simulink model "Target_Control_System"  (R2021b)
settings: Solver=FixedStepDiscrete  StartTime=0.0  StopTime=5  RelTol=1e-3
PreLoadFcn:
  | RTWConfigurationCB('preloadfcn', bdroot);
PostLoadFcn:
  | load('configuration/data_struct.mat');
  | load('configuration/fluxMaps_propMotor.mat');
  | load('configuration/parameterInit_PROP.mat');
  | load('configuration/parameterInit_PUMP.mat');
  | load('configuration/parameterInit_PITCH.mat');
  | load('configuration/parameterInit_TILT.mat');
  | %load('configuration/base_workspace_signal_definition.mat');
  | %load('resolvedatastores_to_baseworkspace_for_faster_simulation.mat');
model workspace (MAT data in the model file):
  SIMULATION_OPTIONS : Simulink.Parameter (value not decoded)
  TARGET_CODE_GEN : Simulink.Parameter (value not decoded)
  TCS_SAMPLE_FREQ_HZ : Simulink.Parameter (value not decoded)
symbols that are objects in the model workspace (value not decoded): TARGET_CODE_GEN, TCS_SAMPLE_FREQ_HZ
undefined symbols (not defined in the file): A_DQ_REF_LPF_INIT__PITCH, A_DQ_REF_LPF_INIT__PROP, A_DQ_REF_LPF_INIT__PUMP, A_DQ_REF_LPF_INIT__TILT, A_OBSERVER_CONFIDENCE_INIT__PITCH, A_OBSERVER_CONFIDENCE_INIT__PROP, A_OBSERVER_CONFIDENCE_INIT__PUMP, A_OBSERVER_CONFIDENCE_INIT__TILT, ACTUATOR_MAX_ANGLE_TRIP__PITCH, ACTUATOR_MIN_ANGLE_TRIP__PITCH, ACTUATOR_POS_SENSOR_INV_DIRECTION__PITCH, ACTUATOR_POS_SENSOR_INV_DIRECTION__TILT, ACTUATOR_POS_SENSOR_OFFSET__PITCH, ACTUATOR_POS_SENSOR_OFFSET__TILT, ADC_scaler1_baseaddr_TILT, ADC_SCALER_FLOAT_TO_FIXPOINT_EXPANSION, ANGLE_ELEC_FROM_SENSOR_OFFSET_INIT__PITCH, ANGLE_ELEC_FROM_SENSOR_OFFSET_INIT__PROP, ANGLE_ELEC_FROM_SENSOR_OFFSET_INIT__PUMP, ANGLE_ELEC_FROM_SENSOR_OFFSET_INIT__TILT, AUTO_CLEAR_FAULTS_ENABLED__PITCH, AUTO_CLEAR_FAULTS_ENABLED__PROP, AUTO_CLEAR_FAULTS_ENABLED__PUMP, AUTO_CLEAR_FAULTS_ENABLED__TILT, AUTO_CLEAR_FAULTS_WAIT_TICKS__PITCH, AUTO_CLEAR_FAULTS_WAIT_TICKS__PROP, AUTO_CLEAR_FAULTS_WAIT_TICKS__PUMP, AUTO_CLEAR_FAULTS_WAIT_TICKS__TILT, AUTO_I_ZERO_IDLE_TICKS__PITCH, AUTO_I_ZERO_IDLE_TICKS__PROP, AUTO_I_ZERO_IDLE_TICKS__PUMP, AUTO_I_ZERO_IDLE_TICKS__TILT, AUTO_I_ZERO_OFFSET_IDC_THRESHOLD__PITCH, AUTO_I_ZERO_OFFSET_IDC_THRESHOLD__PROP, AUTO_I_ZERO_OFFSET_IDC_THRESHOLD__PUMP, AUTO_I_ZERO_OFFSET_IDC_THRESHOLD__TILT, AUTO_I_ZERO_OFFSET_IPH_THRESHOLD__PITCH, AUTO_I_ZERO_OFFSET_IPH_THRESHOLD__PROP, AUTO_I_ZERO_OFFSET_IPH_THRESHOLD__PUMP, AUTO_I_ZERO_OFFSET_IPH_THRESHOLD__TILT, AUTO_SENSORLESS_SWITCHOVER_DISABLE_OMEGA, AUTO_SENSORLESS_SWITCHOVER_ENABLE_OMEGA, AUTO_SENSORLESS_SWITCHOVER_MIN_CONFIDENCE, AUXILIARY_PROTECTION_UNIT_BASEADDR__TILT, blanking_max_error_omega_INIT_PITCH, blanking_max_error_omega_INIT_TILT, blanking_max_error_position_INIT_PITCH, blanking_max_error_position_INIT_TILT, BRUTE_START_I_Q_REF_RAMP_SPEED__PITCH, BRUTE_START_I_Q_REF_RAMP_SPEED__PROP, BRUTE_START_I_Q_REF_RAMP_SPEED__PUMP, BRUTE_START_I_Q_REF_RAMP_SPEED__TILT, CONTROL_LOOP_DT_INIT__PITCH, CONTROL_LOOP_DT_INIT__PROP, CONTROL_LOOP_DT_INIT__PUMP, CONTROL_LOOP_DT_INIT__TILT, CORRECTION_FILTER_SCALE__PITCH, CORRECTION_FILTER_SCALE__PROP, CORRECTION_FILTER_SCALE__PUMP, CORRECTION_FILTER_SCALE__TILT ... (+458)
libraries: simulink x178, Reusables_Lib x24
(part 32 of 47)

== system Target_Control_System/Target_Control_System/Simulation Controls/Simulation Data Store Initialization/setupPwm()/setPwmFrequencyApplication()_pitch/updateObserver()_pitch ==
  oIsr_.oParam_.fControlLoopDt_ : Inport
  fObserverLoopFilterBandwidthHz_ : Inport  Port=2
  Constant : Constant  Value=15*2*pi  OutDataTypeStr=single  SampleTime=-1
  Constant1 : Constant  Value=8*2*pi  OutDataTypeStr=single  SampleTime=-1
  Constant2 : Constant  Value=2*pi  OutDataTypeStr=single  SampleTime=-1
  Constant3 : Constant  Value=500  OutDataTypeStr=single  SampleTime=-1
  Constant4 : Constant  Value=20  OutDataTypeStr=single  SampleTime=-1
  Constant5 : Constant  Value=100*2*pi  OutDataTypeStr=single  SampleTime=-1
  Constant6 : Constant  Value=4*2*pi  OutDataTypeStr=single  SampleTime=-1
  Constant7 : Constant  Value=0.0625  OutDataTypeStr=single  SampleTime=-1
  Data Store Write : DataStoreWrite  DataStoreName=oPitch  DataStoreElements=oPitch.oIsr_.oParam_.fALpf4hpfDcBlocking_  IndexOptions=Index vector (dialog)  Indices=1  OutputSizes=1
  Data Store Write1 : DataStoreWrite  DataStoreName=oPitch  DataStoreElements=oPitch.oIsr_.oParam_.fAFluxMagnitude_  IndexOptions=Index vector (dialog)  Indices=1  OutputSizes=1
  Data Store Write2 : DataStoreWrite  DataStoreName=oPitch  DataStoreElements=oPitch.oIsr_.oParam_.fALoopfilter2_  IndexOptions=Index vector (dialog)  Indices=1  OutputSizes=1
  Data Store Write3 : DataStoreWrite  DataStoreName=oPitch  DataStoreElements=oPitch.oMot_.oParam_.fObserverLoopFilterBandwidthHz_  IndexOptions=Index vector (dialog)  Indices=1  OutputSizes=1
  Data Store Write4 : DataStoreWrite  DataStoreName=oPitch  DataStoreElements=oPitch.oIsr_.oParam_.fAOmegaFilter2_  IndexOptions=Index vector (dialog)  Indices=1  OutputSizes=1
  Data Store Write5 : DataStoreWrite  DataStoreName=oPitch  DataStoreElements=oPitch.oMot_.oParam_.fAOmegaXfilter2_  IndexOptions=Index vector (dialog)  Indices=1  OutputSizes=1
  Data Store Write6 : DataStoreWrite  DataStoreName=oPitch  DataStoreElements=oPitch.oIsr_.oParam_.oPiDataPll2_.oParameter_.fKp_  IndexOptions=Index vector (dialog)  Indices=1  OutputSizes=1
  Divide{,1,3..4} (4 alike) : Product  Inputs=**
  Divide2 : Product  Inputs=***
  Divide5 : Product  Inputs=*/
  GreaterThan : RelationalOperator  Operator=<  OutDataTypeStr=boolean  RndMeth=Simplest
  Saturation{,1..4} (5 alike) : Saturate  UpperLimit=1.0  LowerLimit=1e-6
  Switch : Switch  Criteria=u2 > Threshold
  wires:
  Divide5/1 -> Data Store Write6/1
  Constant7/1 -> Divide5/1
  Saturation4/1 -> Data Store Write5/1
  oIsr_.oParam_.fControlLoopDt_/1 -> Divide/1, Divide1/1, Divide3/1, Divide2/2, Divide5/2, Divide4/1
  Divide4/1 -> Saturation4/1
  Constant6/1 -> Divide4/2
  Saturation3/1 -> Data Store Write4/1
  Divide3/1 -> Saturation3/1
  Constant5/1 -> Divide3/2
  Switch/1 -> Data Store Write3/1, Divide2/1
  Constant3/1 -> Switch/1
  GreaterThan/1 -> Switch/2
  Constant4/1 -> GreaterThan/2
  fObserverLoopFilterBandwidthHz_/1 -> Switch/3, GreaterThan/1
  Divide2/1 -> Saturation2/1
  Saturation2/1 -> Data Store Write2/1
  Constant2/1 -> Divide2/3
  Divide1/1 -> Saturation1/1
  Saturation1/1 -> Data Store Write1/1
  Constant1/1 -> Divide1/2
  Saturation/1 -> Data Store Write/1
  Divide/1 -> Saturation/1
  Constant/1 -> Divide/2

== system Target_Control_System/Target_Control_System/Simulation Controls/Simulation Data Store Initialization/updateServoObserver(&oTilt)/updateServoObserver()/softwareIirFilterInitialize() ==
  fFreq3db : Inport
  fFreqSample : Inport  Port=2  OutDataTypeStr=single
  Constant : Constant  OutDataTypeStr=single  SampleTime=-1
  Constant1 : Constant  Value=0  OutDataTypeStr=single  SampleTime=-1
  Data Store Write : DataStoreWrite  DataStoreName=oTilt  DataStoreElements=oTilt.oMot_.oState_.oPosSensor_.oInputSensorSpeedFilter_.afConstantsA_.h0  IndexOptions=Index vector (dialog)  Indices=1  OutputSizes=1
  Data Store Write1 : DataStoreWrite  DataStoreName=oTilt  DataStoreElements=oTilt.oMot_.oState_.oPosSensor_.oInputSensorSpeedFilter_.afConstantsA_.h1  IndexOptions=Index vector (dialog)  Indices=1  OutputSizes=1
  Data Store Write10 : DataStoreWrite  DataStoreName=oTilt  DataStoreElements=oTilt.oMot_.oState_.oPosSensor_.oInputSensorSpeedFilter_.fFilterOutput_  IndexOptions=Index vector (dialog)  Indices=1  OutputSizes=1
  Data Store Write2 : DataStoreWrite  DataStoreName=oTilt  DataStoreElements=oTilt.oMot_.oState_.oPosSensor_.oInputSensorSpeedFilter_.afConstantsA_.h2  IndexOptions=Index vector (dialog)  Indices=1  OutputSizes=1
  Data Store Write3 : DataStoreWrite  DataStoreName=oTilt  DataStoreElements=oTilt.oMot_.oState_.oPosSensor_.oInputSensorSpeedFilter_.afConstantsB_.h2  IndexOptions=Index vector (dialog)  Indices=1  OutputSizes=1
  Data Store Write4 : DataStoreWrite  DataStoreName=oTilt  DataStoreElements=oTilt.oMot_.oState_.oPosSensor_.oInputSensorSpeedFilter_.afConstantsB_.h1  IndexOptions=Index vector (dialog)  Indices=1  OutputSizes=1
  Data Store Write5 : DataStoreWrite  DataStoreName=oTilt  DataStoreElements=oTilt.oMot_.oState_.oPosSensor_.oInputSensorSpeedFilter_.afConstantsB_.h0  IndexOptions=Index vector (dialog)  Indices=1  OutputSizes=1
  Data Store Write6 : DataStoreWrite  DataStoreName=oTilt  DataStoreElements=oTilt.oMot_.oState_.oPosSensor_.oInputSensorSpeedFilter_.afPreviousInputs_.h0  IndexOptions=Index vector (dialog)  Indices=1  OutputSizes=1
  Data Store Write7 : DataStoreWrite  DataStoreName=oTilt  DataStoreElements=oTilt.oMot_.oState_.oPosSensor_.oInputSensorSpeedFilter_.afPreviousInputs_.h1  IndexOptions=Index vector (dialog)  Indices=1  OutputSizes=1
  Data Store Write8 : DataStoreWrite  DataStoreName=oTilt  DataStoreElements=oTilt.oMot_.oState_.oPosSensor_.oInputSensorSpeedFilter_.afPreviousOutputs_.h0  IndexOptions=Index vector (dialog)  Indices=1  OutputSizes=1
  Data Store Write9 : DataStoreWrite  DataStoreName=oTilt  DataStoreElements=oTilt.oMot_.oState_.oPosSensor_.oInputSensorSpeedFilter_.afPreviousOutputs_.h1  IndexOptions=Index vector (dialog)  Indices=1  OutputSizes=1
  Data Type Conversion{,1..4} (5 alike) : DataTypeConversion  OutDataTypeStr=single
  Demux : Demux  Outputs=6
  Divide : Product  Inputs=*/  OutDataTypeStr=single
  computeCoefficientsButter() : Subsystem
  fActualFrequencyHz : Outport
  wires:
  fFreqSample/1 -> computeCoefficientsButter()/2(dSampleFrequencyHz)
  Data Type Conversion4/1 -> Data Store Write2/1
  Data Type Conversion3/1 -> Data Store Write1/1
  Data Type Conversion2/1 -> Data Store Write3/1
  Data Type Conversion/1 -> Data Store Write4/1
  Data Type Conversion1/1 -> Data Store Write5/1
  Constant1/1 -> Data Store Write6/1, Data Store Write7/1, Data Store Write9/1, Data Store Write10/1, Data Store Write8/1
  Demux/1 -> Data Type Conversion1/1
  Demux/2 -> Data Type Conversion/1
  Constant/1 -> Divide/1
  Divide/1 -> Data Store Write/1
  Demux/4 -> Divide/2
  Demux/3 -> Data Type Conversion2/1
  Demux/5 -> Data Type Conversion3/1
  Demux/6 -> Data Type Conversion4/1
  computeCoefficientsButter()/1(dpOutArray) -> Demux/1
  fFreq3db/1 -> computeCoefficientsButter()/1(fCutoffFrequencyHz)
  computeCoefficientsButter()/2(fFreq3db) -> fActualFrequencyHz/1

== system Target_Control_System/Target_Control_System/Simulation Controls/Simulation Data Store Initialization/updateServoObserver()/updateServoObserver()_pitch/softwareIirFilterInitialize() ==
  fFreq3db : Inport
  fFreqSample : Inport  Port=2  OutDataTypeStr=single
  Constant : Constant  OutDataTypeStr=single  SampleTime=-1
  Constant1 : Constant  Value=0  OutDataTypeStr=single  SampleTime=-1
  Data Store Write : DataStoreWrite  DataStoreName=oPitch  DataStoreElements=oPitch.oMot_.oState_.oPosSensor_.oInputSensorSpeedFilter_.afConstantsA_.h0  IndexOptions=Index vector (dialog)  Indices=1  OutputSizes=1
  Data Store Write1 : DataStoreWrite  DataStoreName=oPitch  DataStoreElements=oPitch.oMot_.oState_.oPosSensor_.oInputSensorSpeedFilter_.afConstantsA_.h1  IndexOptions=Index vector (dialog)  Indices=1  OutputSizes=1
  Data Store Write10 : DataStoreWrite  DataStoreName=oPitch  DataStoreElements=oPitch.oMot_.oState_.oPosSensor_.oInputSensorSpeedFilter_.fFilterOutput_  IndexOptions=Index vector (dialog)  Indices=1  OutputSizes=1
  Data Store Write2 : DataStoreWrite  DataStoreName=oPitch  DataStoreElements=oPitch.oMot_.oState_.oPosSensor_.oInputSensorSpeedFilter_.afConstantsA_.h2  IndexOptions=Index vector (dialog)  Indices=1  OutputSizes=1
  Data Store Write3 : DataStoreWrite  DataStoreName=oPitch  DataStoreElements=oPitch.oMot_.oState_.oPosSensor_.oInputSensorSpeedFilter_.afConstantsB_.h2  IndexOptions=Index vector (dialog)  Indices=1  OutputSizes=1
  Data Store Write4 : DataStoreWrite  DataStoreName=oPitch  DataStoreElements=oPitch.oMot_.oState_.oPosSensor_.oInputSensorSpeedFilter_.afConstantsB_.h1  IndexOptions=Index vector (dialog)  Indices=1  OutputSizes=1
  Data Store Write5 : DataStoreWrite  DataStoreName=oPitch  DataStoreElements=oPitch.oMot_.oState_.oPosSensor_.oInputSensorSpeedFilter_.afConstantsB_.h0  IndexOptions=Index vector (dialog)  Indices=1  OutputSizes=1
  Data Store Write6 : DataStoreWrite  DataStoreName=oPitch  DataStoreElements=oPitch.oMot_.oState_.oPosSensor_.oInputSensorSpeedFilter_.afPreviousInputs_.h0  IndexOptions=Index vector (dialog)  Indices=1  OutputSizes=1
  Data Store Write7 : DataStoreWrite  DataStoreName=oPitch  DataStoreElements=oPitch.oMot_.oState_.oPosSensor_.oInputSensorSpeedFilter_.afPreviousInputs_.h1  IndexOptions=Index vector (dialog)  Indices=1  OutputSizes=1
  Data Store Write8 : DataStoreWrite  DataStoreName=oPitch  DataStoreElements=oPitch.oMot_.oState_.oPosSensor_.oInputSensorSpeedFilter_.afPreviousOutputs_.h0  IndexOptions=Index vector (dialog)  Indices=1  OutputSizes=1
  Data Store Write9 : DataStoreWrite  DataStoreName=oPitch  DataStoreElements=oPitch.oMot_.oState_.oPosSensor_.oInputSensorSpeedFilter_.afPreviousOutputs_.h1  IndexOptions=Index vector (dialog)  Indices=1  OutputSizes=1
  Data Type Conversion{,1..4} (5 alike) : DataTypeConversion  OutDataTypeStr=single
  Demux : Demux  Outputs=6
  Divide : Product  Inputs=*/  OutDataTypeStr=single
  computeCoefficientsButter() : Subsystem
  fActualFrequencyHz : Outport
  wires:
  fFreqSample/1 -> computeCoefficientsButter()/2(dSampleFrequencyHz)
  Data Type Conversion4/1 -> Data Store Write2/1
  Data Type Conversion3/1 -> Data Store Write1/1
  Data Type Conversion2/1 -> Data Store Write3/1
  Data Type Conversion/1 -> Data Store Write4/1
  Data Type Conversion1/1 -> Data Store Write5/1
  Constant1/1 -> Data Store Write6/1, Data Store Write7/1, Data Store Write9/1, Data Store Write10/1, Data Store Write8/1
  Demux/1 -> Data Type Conversion1/1
  Demux/2 -> Data Type Conversion/1
  Constant/1 -> Divide/1
  Divide/1 -> Data Store Write/1
  Demux/4 -> Divide/2
  Demux/3 -> Data Type Conversion2/1
  Demux/5 -> Data Type Conversion3/1
  Demux/6 -> Data Type Conversion4/1
  computeCoefficientsButter()/1(dpOutArray) -> Demux/1
  fFreq3db/1 -> computeCoefficientsButter()/1(fCutoffFrequencyHz)
  computeCoefficientsButter()/2(fFreq3db) -> fActualFrequencyHz/1

== system Target_Control_System/Target_Control_System/InterruptFunction/pitchMotor_dataToMain/Variant Subsystem/VP_leader_follower_postion_copy/Follower Postion Enabled Subsystem/System Update ==

== system Target_Control_System/Target_Control_System/InterruptFunction/pitchMotor_dataToMain/Variant Subsystem/VP_leader_follower_postion_copy/Leader Postion Enabled Subsystem/System Update ==

== system Target_Control_System/Target_Control_System/InterruptFunction/pitchMotor_isrTask/abcToAlphaBeta/ModelSource/IncludeCustomCode/System Update ==

== system Target_Control_System/Target_Control_System/InterruptFunction/pitchMotor_isrTask/currentController/Current Controller/Limit Voltage Vector/Compute Alpha-Beta Refs ==
  In1 : Inport
  Out1 : Outport
  wires:
  In1/1 -> Out1/1

== system Target_Control_System/Target_Control_System/InterruptFunction/pitchMotor_isrTask/fluxAngleCalculations/ModelSource/IncludeCustomCode/System Update ==

== system Target_Control_System/Target_Control_System/InterruptFunction/propMotor_isrTask/abcToAlphaBeta/ModelSourceFOProp/IncludeCustomCode/System Update ==

== system Target_Control_System/Target_Control_System/InterruptFunction/propMotor_isrTask/currentController/Subsystem/Limit Voltage Vector/Subsystem ==
  fMaximumVoltageVectorLengthSquared_ : Inport
  UdRef*UdRef : Inport  Port=2
  In3 : Inport  Port=3
  Enable : EnablePort
  Add1 : Sum  Inputs=+-
  Constant1 : Constant  Value=0  OutDataTypeStr=single  SampleTime=-1
  Divide3 : Product  Inputs=**
  Max : MinMax  Function=max  Inputs=2
  Sqrt : Sqrt  SaturateOnIntegerOverflow=on
  Out1 : Outport
  wires:
  UdRef*UdRef/1 -> Add1/2
  fMaximumVoltageVectorLengthSquared_/1 -> Add1/1
  Divide3/1 -> Out1/1
  Add1/1 -> Max/2
  Constant1/1 -> Max/1
  Max/1 -> Sqrt/1
  In3/1 -> Divide3/2
  Sqrt/1 -> Divide3/1

== system Target_Control_System/Target_Control_System/InterruptFunction/propMotor_isrTask/fluxAngleCalculation/ModelSource/IncludeCustomCode/System Update ==

== system Target_Control_System/Target_Control_System/InterruptFunction/pumpMotor_isrTask/abcToAlphaBeta/ModelSource/IncludeCustomCode/System Update ==

== system Target_Control_System/Target_Control_System/InterruptFunction/pumpMotor_isrTask/currentController/Subsystem/Limit Voltage Vector/Subsystem ==
  fMaximumVoltageVectorLengthSquared_ : Inport
  UdRef*UdRef : Inport  Port=2
  In3 : Inport  Port=3
  Enable : EnablePort
  Add1 : Sum  Inputs=+-
  Constant1 : Constant  Value=0  OutDataTypeStr=single  SampleTime=-1
  Divide3 : Product  Inputs=**
  Max : MinMax  Function=max  Inputs=2
  Sqrt : Sqrt  SaturateOnIntegerOverflow=on
  Out1 : Outport
  wires:
  UdRef*UdRef/1 -> Add1/2
  fMaximumVoltageVectorLengthSquared_/1 -> Add1/1
  Divide3/1 -> Out1/1
  Add1/1 -> Max/2
  Constant1/1 -> Max/1
  Max/1 -> Sqrt/1
  In3/1 -> Divide3/2
  Sqrt/1 -> Divide3/1

== system Target_Control_System/Target_Control_System/InterruptFunction/pumpMotor_isrTask/fluxAngleCalculations/ModelSource1/IncludeCustomCode/System Update ==

== system Target_Control_System/Target_Control_System/InterruptFunction/tiltMotor_isrTask/abcToAlphaBeta/ModelSource/IncludeCustomCode/System Update ==

== system Target_Control_System/Target_Control_System/InterruptFunction/tiltMotor_isrTask/currentController/Enabled Subsystem/Limit Voltage Vector/Compute Alpha-Beta Refs ==
  In1 : Inport
  Out1 : Outport
  wires:
  In1/1 -> Out1/1

== system Target_Control_System/Target_Control_System/InterruptFunction/tiltMotor_isrTask/fluxAngleCalculation/ModelSource/IncludeCustomCode/System Update ==

== system Target_Control_System/Target_Control_System/MainLoop/pitchMotor_mainLoop/Decimation gate for 10 Hz Pitch/Function-Call Subsystem/Dynamic_current_limiting_pitch/Enabled Subsystem ==
  Enable : EnablePort
  Constant : Constant  Value=0  OutDataTypeStr=single  SampleTime=-1
  Constant1 : Constant  Value=200  OutDataTypeStr=single  SampleTime=-1
  Constant3 : Constant  Value=0  OutDataTypeStr=single  SampleTime=-1
  Data Store Read : DataStoreRead  DataStoreName=oPitch  DataStoreElements=oPitch.oMot_.oParam_.fDynILimDynamicMax_  IndexOptions=Index vector (dialog)  Indices=1  OutputSizes=1
  Data Store Read1 : DataStoreRead  DataStoreName=oPitch  DataStoreElements=oPitch.oMot_.oParam_.fDynILimKnockdownFactor_  IndexOptions=Index vector (dialog)  Indices=1  OutputSizes=1
  Data Store Read2 : DataStoreRead  DataStoreName=oPitch  DataStoreElements=oPitch.oMot_.oParam_.fDynILimDynamicMax_  IndexOptions=Index vector (dialog)  Indices=1  OutputSizes=1
  Data Store Read3 : DataStoreRead  DataStoreName=oPitch  DataStoreElements=oPitch.oMot_.oState_.fDynILimIntegrator_  IndexOptions=Index vector (dialog)  Indices=1  OutputSizes=1
  Data Store Read4 : DataStoreRead  DataStoreName=oPitch  DataStoreElements=oPitch.oMot_.oParam_.oPiDataRpm_.oParameter_.fOutMin_  IndexOptions=Index vector (dialog)  Indices=1  OutputSizes=1
  Data Store Read5 : DataStoreRead  DataStoreName=oPitch  DataStoreElements=oPitch.oMot_.oState_.fDynILimActualLimit_  IndexOptions=Index vector (dialog)  Indices=1  OutputSizes=1
  Data Store Read6 : DataStoreRead  DataStoreName=oPitch  DataStoreElements=oPitch.oMot_.oParam_.oPiDataRpm_.oParameter_.fIntMin_  IndexOptions=Index vector (dialog)  Indices=1  OutputSizes=1
  Data Store Read7 : DataStoreRead  DataStoreName=oPitch  DataStoreElements=oPitch.oMot_.oState_.uiDriveState_  IndexOptions=Index vector (dialog)  Indices=1  OutputSizes=1
  Data Store Write : DataStoreWrite  DataStoreName=oTilt  DataStoreElements=oTilt.oMot_.oState_.fDynILimIntegrator_  IndexOptions=Index vector (dialog)  Indices=1  OutputSizes=1
  Data Store Write1 : DataStoreWrite  DataStoreName=oTilt  DataStoreElements=oTilt.oMot_.oParam_.oPiDataRpm_.oParameter_.fOutMax_  IndexOptions=Index vector (dialog)  Indices=1  OutputSizes=1
  Data Store Write2 : DataStoreWrite  DataStoreName=oTilt  DataStoreElements=oTilt.oMot_.oParam_.oPiDataRpm_.oParameter_.fOutMin_  IndexOptions=Index vector (dialog)  Indices=1  OutputSizes=1
  Data Store Write3 : DataStoreWrite  DataStoreName=oTilt  DataStoreElements=oTilt.oMot_.oParam_.oPiDataRpm_.oParameter_.fIntMin_  IndexOptions=Index vector (dialog)  Indices=1  OutputSizes=1
  Data Store Write4 : DataStoreWrite  DataStoreName=oTilt  DataStoreElements=oTilt.oMot_.oParam_.oPiDataRpm_.oParameter_.fIntMax_  IndexOptions=Index vector (dialog)  Indices=1  OutputSizes=1
  Divide : Product  Inputs=*/
  Enabled Subsystem : Subsystem  TreatAsAtomicUnit=on
  Gain : Gain  Gain=3
  IsNaN : RelationalOperator  Operator=isNaN  OutDataTypeStr=boolean  RndMeth=Simplest
  Less Than : RelationalOperator  Operator=<  OutDataTypeStr=boolean  RndMeth=Simplest
  Saturation Dynamic : simulink/Discontinuities/Saturation Dynamic  OutMin=[]  OutMax=[]  OutDataTypeStr=Inherit: Same as second input  OutDataType=fixdt(1, 16)  OutScaling=2^-10  DoSatur=off
  Switch : Switch  Criteria=u2 > Threshold
  Switch2 : Switch  Criteria=u2 > Threshold
  Switch3 : Switch  Criteria=u2 > Threshold
  Unary Minus : UnaryMinus
  Unary Minus1 : UnaryMinus
  wires:
  Data Store Read2/1 -> Data Store Write1/1, Unary Minus/1
  Less Than/1 -> Enabled Subsystem/Enable
  Unary Minus/1 -> Switch2/1
  Data Store Read3/1 -> IsNaN/1, Switch/3
  Data Store Read5/1 -> Data Store Write4/1, Unary Minus1/1
  Gain/1 -> Saturation Dynamic/1
  Constant1/1 -> Less Than/2
  Constant3/1 -> Saturation Dynamic/3
  Switch3/1 -> Data Store Write3/1
  Switch2/1 -> Data Store Write2/1
  Unary Minus1/1 -> Switch3/1
  Data Store Read/1 -> Divide/1
  Data Store Read4/1 -> Switch2/3, Switch2/2
  Data Store Read7/1 -> Less Than/1
  Divide/1 -> Gain/1
  Data Store Read1/1 -> Divide/2
  Saturation Dynamic/1 -> Data Store Write/1  "fDynLimIntegrator"
  IsNaN/1 -> Switch/2
  Switch/1 -> Saturation Dynamic/2
  Data Store Read6/1 -> Switch3/3, Switch3/2
  Constant/1 -> Switch/1

== system Target_Control_System/Target_Control_System/MainLoop/pitchMotor_mainLoop/Decimation gate for 200 Hz Pitch/Function-Call Subsystem/Check zero current if inverter off/Enabled Subsystem ==
  note: The inverter is idle (mosfets are off), and the current sensors have been offset corrected.
      | The current sensor readings should be fairly close to zero.
  Enable : EnablePort
  Chart : Stateflow chart  TreatAsAtomicUnit=on

== system Target_Control_System/Target_Control_System/MainLoop/pitchMotor_mainLoop/Decimation gate for 200 Hz Pitch/Function-Call Subsystem/Current control inactive/Enabled Subsystem ==
  note: Keep the speed controller integrator value at zero
  Enable : EnablePort
  Constant : Constant  Value=0  OutDataTypeStr=single  SampleTime=-1
  Data Store Write : DataStoreWrite  DataStoreName=oPitch  DataStoreElements=oPitch.oMot_.oParam_.oPiDataRpm_.fState_  IndexOptions=Index vector (dialog)  Indices=1  OutputSizes=1
  Data Store Write1 : DataStoreWrite  DataStoreName=oPitch  DataStoreElements=oPitch.oMot_.oParam_.oPid2DataRpmCtrl_.fState_  IndexOptions=Index vector (dialog)  Indices=1  OutputSizes=1
  wires:
  Constant/1 -> Data Store Write/1, Data Store Write1/1

== system Target_Control_System/Target_Control_System/MainLoop/pitchMotor_mainLoop/Decimation gate for 200 Hz Pitch/Function-Call Subsystem/Current offset nulling/initiateOffsetNulling(&oPitch) ==
  note: Further checks for starting the nulling process are handled inside the lower level function
  Enable : EnablePort
  Chart : Stateflow chart  TreatAsAtomicUnit=on

== system Target_Control_System/Target_Control_System/MainLoop/pitchMotor_mainLoop/Decimation gate for 200 Hz Pitch/Function-Call Subsystem/Forced current injection for broken input sensors/Enabled Subsystem ==
  note: Forced current injection for broken input position sensors:
      | 226 = a signaling state, the inverter is not actually on
      | 227 = the actual on state, pure 0 RPM
      | 228 = rudimentary position control using only the output position sensor
  Enable : EnablePort
  Constant : Constant  OutDataTypeStr=uint32  SampleTime=-1
  Constant1 : Constant  Value=0  OutDataTypeStr=int32  SampleTime=-1
  Constant2 : Constant  Value=0  OutDataTypeStr=uint32  SampleTime=-1
  Constant3 : Constant  Value=228  OutDataTypeStr=uint32  SampleTime=-1
  Data Store Read : DataStoreRead  DataStoreName=oPitch  DataStoreElements=oPitch.oMot_.oState_.uiDriveState_  IndexOptions=Index vector (dialog)  Indices=1  OutputSizes=1
  Data Store Write : DataStoreWrite  DataStoreName=oPitch  DataStoreElements=oPitch.oMot_.oOut_.uiForcedAngle_  IndexOptions=Index vector (dialog)  Indices=1  OutputSizes=1
  Data Store Write1 : DataStoreWrite  DataStoreName=oPitch  DataStoreElements=oPitch.oMot_.oState_.oPosSensor_.iPosControlEnabled_  IndexOptions=Index vector (dialog)  Indices=1  OutputSizes=1
  Data Store Write2 : DataStoreWrite  DataStoreName=oPitch  DataStoreElements=oPitch.oMot_.oState_.uiSpeedControllerActive_  IndexOptions=Index vector (dialog)  Indices=1  OutputSizes=1
  NOT : Logic  Operator=NOT  IconShape=distinctive  AllPortsSameDT=off  OutDataTypeStr=boolean
  NotEqual : RelationalOperator  Operator=~=  OutDataTypeStr=boolean  RndMeth=Simplest
  Pure_0rpm_holding_mode : Subsystem  TreatAsAtomicUnit=on
  Rudimentary_forced_angle_position_control : Subsystem  TreatAsAtomicUnit=on
  wires:
  NOT/1 -> Rudimentary_forced_angle_position_control/Enable
  NotEqual/1 -> Pure_0rpm_holding_mode/Enable, NOT/1
  Constant3/1 -> NotEqual/2
  Data Store Read/1 -> NotEqual/1
  Constant2/1 -> Data Store Write2/1
  Constant1/1 -> Data Store Write1/1
  Constant/1 -> Data Store Write/1

== system Target_Control_System/Target_Control_System/MainLoop/pitchMotor_mainLoop/Decimation gate for 200 Hz Pitch/Function-Call Subsystem/Idle controller/Forced angle ==
  Enable : EnablePort
  Data Store Write : DataStoreWrite  DataStoreName=oPitch  DataStoreElements=oPitch.oMot_.oParam_.oPiDataIdleCtrl_.fState_  IndexOptions=Index vector (dialog)  Indices=1  OutputSizes=1
  Data Store Write11 : DataStoreWrite  DataStoreName=oPitch  DataStoreElements=oPitch.oMot_.oState_.fIdleCtrlCurrent_  IndexOptions=Index vector (dialog)  Indices=1  OutputSizes=1
  Zero16 : Constant  Value=0  OutDataTypeStr=single  SampleTime=-1
  wires:
  Zero16/1 -> Data Store Write/1, Data Store Write11/1

== system Target_Control_System/Target_Control_System/MainLoop/pitchMotor_mainLoop/Decimation gate for 200 Hz Pitch/Function-Call Subsystem/Idle controller/Not forced angle ==
  Enable : EnablePort
  Data Store Read1 : DataStoreRead  DataStoreName=oPitch  DataStoreElements=oPitch.oMot_.oParam_.oPiDataIdleCtrl_.oParameter_.fIntMin_  IndexOptions=Index vector (dialog)  Indices=1  OutputSizes=1
  Data Store Read2 : DataStoreRead  DataStoreName=oPitch  DataStoreElements=oPitch.oMot_.oParam_.oPiDataIdleCtrl_.oParameter_.fOutMin_  IndexOptions=Index vector (dialog)  Indices=1  OutputSizes=1
  Data Store Read3 : DataStoreRead  DataStoreName=oPitch  DataStoreElements=oPitch.oMot_.oParam_.oPiDataIdleCtrl_.fState_  IndexOptions=Index vector (dialog)  Indices=1  OutputSizes=1
  Data Store Read65 : DataStoreRead  DataStoreName=oPitch  DataStoreElements=oPitch.oMot_.oOut_.fOmegaEObserverXlpf2_  IndexOptions=Index vector (dialog)  Indices=1  OutputSizes=1
  Data Store Read66 : DataStoreRead  DataStoreName=oPitch  DataStoreElements=oPitch.oMot_.oState_.fIdleCtrlOmegaEMin_  IndexOptions=Index vector (dialog)  Indices=1  OutputSizes=1
  Data Store Read67 : DataStoreRead  DataStoreName=oPitch  DataStoreElements=oPitch.oMot_.oParam_.oPiDataIdleCtrl_.oParameter_.fKp_  IndexOptions=Index vector (dialog)  Indices=1  OutputSizes=1
  Data Store Read69 : DataStoreRead  DataStoreName=oPitch  DataStoreElements=oPitch.oMot_.oParam_.oPiDataIdleCtrl_.oParameter_.fKi_  IndexOptions=Index vector (dialog)  Indices=1  OutputSizes=1
  Data Store Read70 : DataStoreRead  DataStoreName=oPitch  DataStoreElements=oPitch.oMot_.oParam_.oPiDataIdleCtrl_.oParameter_.fIntMax_  IndexOptions=Index vector (dialog)  Indices=1  OutputSizes=1
  Data Store Read94 : DataStoreRead  DataStoreName=oPitch  DataStoreElements=oPitch.oMot_.oParam_.oPiDataIdleCtrl_.oParameter_.fOutMax_  IndexOptions=Index vector (dialog)  Indices=1  OutputSizes=1
  Data Store Read95 : DataStoreRead  DataStoreName=oPitch  DataStoreElements=oPitch.oMot_.oParam_.oPiDataIdleCtrl_.oParameter_.fLoopDt_  IndexOptions=Index vector (dialog)  Indices=1  OutputSizes=1
  Data Store Write1 : DataStoreWrite  DataStoreName=oPitch  DataStoreElements=oPitch.oMot_.oState_.fIdleCtrlCurrent_  IndexOptions=Index vector (dialog)  Indices=1  OutputSizes=1
  Data Store Write2 : DataStoreWrite  DataStoreName=oPitch  DataStoreElements=oPitch.oMot_.oParam_.oPiDataIdleCtrl_.fState_  IndexOptions=Index vector (dialog)  Indices=1  OutputSizes=1
  Zero19 : Constant  OutDataTypeStr=single  SampleTime=-1
  piControllerStep_Idle_Controller(&oPitch) : Subsystem  SystemSampleTime=1/200
  wires:
  Data Store Read3/1 -> piControllerStep_Idle_Controller(&oPitch)/11(fState)
  piControllerStep_Idle_Controller(&oPitch)/2(*fpState) -> Data Store Write2/1
  piControllerStep_Idle_Controller(&oPitch)/1(fOutput) -> Data Store Write1/1
  Data Store Read2/1 -> piControllerStep_Idle_Controller(&oPitch)/10(fOutMin)
  Data Store Read94/1 -> piControllerStep_Idle_Controller(&oPitch)/8(fOutMax)
  Data Store Read1/1 -> piControllerStep_Idle_Controller(&oPitch)/9(fIntMin)
  Zero19/1 -> piControllerStep_Idle_Controller(&oPitch)/5(fScale)
  Data Store Read70/1 -> piControllerStep_Idle_Controller(&oPitch)/7(fIntMax)
  Data Store Read95/1 -> piControllerStep_Idle_Controller(&oPitch)/6(fLoopDt)
  Data Store Read65/1 -> piControllerStep_Idle_Controller(&oPitch)/1(fActual)
  Data Store Read67/1 -> piControllerStep_Idle_Controller(&oPitch)/3(fKp)
  Data Store Read66/1 -> piControllerStep_Idle_Controller(&oPitch)/2(fTarget)
  Data Store Read69/1 -> piControllerStep_Idle_Controller(&oPitch)/4(fKi)

== system Target_Control_System/Target_Control_System/MainLoop/pitchMotor_mainLoop/Decimation gate for 200 Hz Pitch/Function-Call Subsystem/Position control checks/NOT position control mode ==
  note: Not in position control mode, so either torque or speed mode (=prop and pumpfan)
      | Evaluate need for blanking (with hysteresis if the confidence is inbetween):
  Enable : EnablePort
  Chart : Stateflow chart  TreatAsAtomicUnit=on

== system Target_Control_System/Target_Control_System/MainLoop/pitchMotor_mainLoop/Decimation gate for 200 Hz Pitch/Function-Call Subsystem/Position control checks/Position control mode ==
  Enable : EnablePort
  Check AD2S1210 : Subsystem  Commented=on  TreatAsAtomicUnit=on
  Check fighting controllers : Subsystem  TreatAsAtomicUnit=on
  Check for position halted : Subsystem  TreatAsAtomicUnit=on
  Function-Call Generator : simulink/Ports & Subsystems/Function-Call Generator  sample_time=-1  numberOfIterations=1  DisallowWideOutput=off
  Function-Call Split1 : FunctionCallSplit  NumOutputPorts=2
  Function-Call Split10 : FunctionCallSplit  NumOutputPorts=2
  Function-Call Split2 : FunctionCallSplit  NumOutputPorts=2
  checkSensorLimits(&oPitch) : Subsystem  TreatAsAtomicUnit=on
  wires:
  Function-Call Split2/2 -> Check fighting controllers/Trigger
  Function-Call Split2/1 -> Check AD2S1210/Trigger
  Function-Call Split1/2 -> Function-Call Split2/1
  Function-Call Split1/1 -> checkSensorLimits(&oPitch)/Trigger
  Function-Call Split10/2 -> Function-Call Split1/1
  Function-Call Split10/1 -> Check for position halted/Trigger
  Function-Call Generator/1 -> Function-Call Split10/1

== system Target_Control_System/Target_Control_System/MainLoop/pitchMotor_mainLoop/Decimation gate for 5000 Hz Pitch/motorTaskProcessExternalSetpoints(&oPitch)/hot_standby/Subsystem ==
  Enable : EnablePort
  Data Store Write19 : DataStoreWrite  DataStoreName=oPitch  DataStoreElements=oPitch.oMot_.oIn_.fIqSetpoint_  IndexOptions=Index vector (dialog)  Indices=1  OutputSizes=1
  const1 : Constant  Value=0.0  OutDataTypeStr=single  SampleTime=-1
  wires:
  const1/1 -> Data Store Write19/1

== system Target_Control_System/Target_Control_System/MainLoop/pitchMotor_mainLoop/Decimation gate for 5000 Hz Pitch/motorTaskProcessExternalSetpoints(&oPitch)/passive_holding_mode/Subsystem ==
  Enable : EnablePort
  Data Store Read68 : DataStoreRead  DataStoreName=oPitch  DataStoreElements=oPitch.oMot_.oParam_.fDynILimDynamicMax_  IndexOptions=Index vector (dialog)  Indices=1  OutputSizes=1
  Data Store Write19 : DataStoreWrite  DataStoreName=oPitch  DataStoreElements=oPitch.oMot_.oIn_.fIqSetpoint_  IndexOptions=Index vector (dialog)  Indices=1  OutputSizes=1
  wires:
  Data Store Read68/1 -> Data Store Write19/1

== system Target_Control_System/Target_Control_System/MainLoop/pitchMotor_mainLoop/Decimation gate for 5000 Hz Pitch/motorTaskProcessExternalSetpoints(&oPitch)/set_target/Id_target ==
  Enable : EnablePort
  AND1 : Logic  Operator=OR  AllPortsSameDT=off  OutDataTypeStr=boolean
  Data Store Read1 : DataStoreRead  DataStoreName=oPitch  DataStoreElements=oPitch.oMot_.oIn_.fIdSetpoint_  IndexOptions=Index vector (dialog)  Indices=1  OutputSizes=1
  IsNaN : RelationalOperator  Operator=isNaN  OutDataTypeStr=boolean  RndMeth=Simplest
  IsNaN1 : RelationalOperator  Operator=isInf  OutDataTypeStr=boolean  RndMeth=Simplest
  NOT1 : Logic  Operator=NOT  AllPortsSameDT=off  OutDataTypeStr=boolean
  Subsystem : Subsystem
  wires:
  NOT1/1 -> AND1/1
  Data Store Read1/1 -> IsNaN1/1, Subsystem/1(Input), IsNaN/1
  IsNaN1/1 -> AND1/2
  IsNaN/1 -> NOT1/1
  AND1/1 -> Subsystem/Enable

== system Target_Control_System/Target_Control_System/MainLoop/pitchMotor_mainLoop/Decimation gate for 5000 Hz Pitch/motorTaskProcessExternalSetpoints(&oPitch)/set_target/Id_zero_for_forced_angle ==
  Enable : EnablePort
  Data Store Write1 : DataStoreWrite  DataStoreName=oPitch  DataStoreElements=oPitch.oMot_.oState_.fIdExternalSetpoint_  IndexOptions=Index vector (dialog)  Indices=1  OutputSizes=1
  Data Store Write19 : DataStoreWrite  DataStoreName=oPitch  DataStoreElements=oPitch.oMot_.oState_.oRampDataIdRef_.fSetpoint_  IndexOptions=Index vector (dialog)  Indices=1  OutputSizes=1
  const1 : Constant  Value=0.0  OutDataTypeStr=single  SampleTime=-1
  wires:
  const1/1 -> Data Store Write19/1, Data Store Write1/1

== system Target_Control_System/Target_Control_System/MainLoop/pitchMotor_mainLoop/Decimation gate for 5000 Hz Pitch/motorTaskProcessExternalSetpoints(&oPitch)/set_target/Iq_target ==
  Enable : EnablePort
  AND : Logic  AllPortsSameDT=off  OutDataTypeStr=boolean
  AND1 : Logic  AllPortsSameDT=off  OutDataTypeStr=boolean
  Data Store Read1 : DataStoreRead  DataStoreName=oPitch  DataStoreElements=oPitch.oMot_.oState_.uiSpeedControllerActive_  IndexOptions=Index vector (dialog)  Indices=1  OutputSizes=1
  Data Store Read2 : DataStoreRead  DataStoreName=oPitch  DataStoreElements=oPitch.oMot_.oState_.oPosSensor_.iPosControlEnabled_  IndexOptions=Index vector (dialog)  Indices=1  OutputSizes=1
  Data Store Read68 : DataStoreRead  DataStoreName=oPitch  DataStoreElements=oPitch.oMot_.oIn_.fIqSetpoint_  IndexOptions=Index vector (dialog)  Indices=1  OutputSizes=1
  Data Store Read85 : DataStoreRead  DataStoreName=oPitch  DataStoreElements=oPitch.oMot_.oParam_.uiTorqueMirroringActive_  IndexOptions=Index vector (dialog)  Indices=1  OutputSizes=1
  IsNaN : RelationalOperator  Operator=isNaN  OutDataTypeStr=boolean  RndMeth=Simplest
  NOT : Logic  Operator=NOT  AllPortsSameDT=off  OutDataTypeStr=boolean
  NOT1 : Logic  Operator=NOT  AllPortsSameDT=off  OutDataTypeStr=boolean
  NOT2 : Logic  Operator=NOT  AllPortsSameDT=off  OutDataTypeStr=boolean
  OR : Logic  Operator=OR  AllPortsSameDT=off  OutDataTypeStr=boolean
  Subsystem : Subsystem
  wires:
  AND1/1 -> Subsystem/Enable
  Data Store Read85/1 -> OR/1
  Data Store Read1/1 -> NOT/1
  AND/1 -> OR/2
  NOT/1 -> AND/1
  Data Store Read2/1 -> NOT1/1
  NOT1/1 -> AND/2
  OR/1 -> AND1/1
  Data Store Read68/1 -> IsNaN/1
  IsNaN/1 -> NOT2/1
  NOT2/1 -> AND1/2

== system Target_Control_System/Target_Control_System/MainLoop/pitchMotor_mainLoop/Decimation gate for 5000 Hz Pitch/motorTaskProcessExternalSetpoints(&oPitch)/set_target/position_target ==
  Enable : EnablePort
  AND : Logic  Operator=OR  AllPortsSameDT=off  OutDataTypeStr=boolean
  AND1 : Logic  Inputs=3  AllPortsSameDT=off  OutDataTypeStr=boolean
  Data Store Read1 : DataStoreRead  DataStoreName=oPitch  DataStoreElements=oPitch.oMot_.oState_.oPosSensor_.iPosControlEnabled_  IndexOptions=Index vector (dialog)  Indices=1  OutputSizes=1
  Data Store Read68 : DataStoreRead  DataStoreName=oPitch  DataStoreElements=oPitch.oMot_.oIn_.fPosSetpoint_  IndexOptions=Index vector (dialog)  Indices=1  OutputSizes=1
  Data Store Read85 : DataStoreRead  DataStoreName=oPitch  DataStoreElements=oPitch.oMot_.oState_.uiDriveState_  IndexOptions=Index vector (dialog)  Indices=1  OutputSizes=1
  Equal1 : RelationalOperator  Operator=~=  OutDataTypeStr=boolean  RndMeth=Simplest
  Equal13 : RelationalOperator  Operator===  OutDataTypeStr=boolean  RndMeth=Simplest
  IsNaN : RelationalOperator  Operator=isNaN  OutDataTypeStr=boolean  RndMeth=Simplest
  NOT2 : Logic  Operator=NOT  AllPortsSameDT=off  OutDataTypeStr=boolean
  Subsystem : Subsystem
  const1 : Constant  Value=202  OutDataTypeStr=uint32  SampleTime=-1
  const17 : Constant  Value=228  OutDataTypeStr=uint32  SampleTime=-1
  wires:
  NOT2/1 -> AND1/3
  const1/1 -> Equal1/2
  Equal1/1 -> AND1/2
  const17/1 -> Equal13/1
  Data Store Read85/1 -> Equal1/1, Equal13/2
  Equal13/1 -> AND/2
  AND/1 -> AND1/1
  Data Store Read1/1 -> AND/1
  IsNaN/1 -> NOT2/1
  Data Store Read68/1 -> IsNaN/1
  AND1/1 -> Subsystem/Enable

== system Target_Control_System/Target_Control_System/MainLoop/pitchMotor_mainLoop/Decimation gate for 5000 Hz Pitch/motorTaskProcessExternalSetpoints(&oPitch)/set_target/speed_target ==
  Enable : EnablePort
  AND1 : Logic  Inputs=3  AllPortsSameDT=off  OutDataTypeStr=boolean
  Data Store Read1 : DataStoreRead  DataStoreName=oPitch  DataStoreElements=oPitch.oMot_.oState_.oPosSensor_.iPosControlEnabled_  IndexOptions=Index vector (dialog)  Indices=1  OutputSizes=1
  Data Store Read2 : DataStoreRead  DataStoreName=oPitch  DataStoreElements=oPitch.oMot_.oParam_.uiAutomaticFanControlMode_  IndexOptions=Index vector (dialog)  Indices=1  OutputSizes=1
  Data Store Read85 : DataStoreRead  DataStoreName=oPitch  DataStoreElements=oPitch.oMot_.oState_.uiDriveState_  IndexOptions=Index vector (dialog)  Indices=1  OutputSizes=1
  Equal13 : RelationalOperator  Operator=~=  OutDataTypeStr=boolean  RndMeth=Simplest
  NOT1 : Logic  Operator=NOT  AllPortsSameDT=off  OutDataTypeStr=boolean
  NOT2 : Logic  Operator=NOT  AllPortsSameDT=off  OutDataTypeStr=boolean
  Subsystem : Subsystem
  const17 : Constant  Value=228  OutDataTypeStr=uint32  SampleTime=-1
  wires:
  Data Store Read2/1 -> NOT2/1
  NOT2/1 -> AND1/2
  const17/1 -> Equal13/1
  Data Store Read85/1 -> Equal13/2
  Equal13/1 -> AND1/3
  NOT1/1 -> AND1/1
  Data Store Read1/1 -> NOT1/1
  AND1/1 -> Subsystem/Enable

== system Target_Control_System/Target_Control_System/MainLoop/pitchMotor_mainLoop/mainTask_pitch/PWM for Simulation/Subsystem1/Subsystem ==
  Enable : EnablePort
  Bus Creator2 : BusCreator  Inputs=3
  Data Store Read2 : DataStoreRead  DataStoreName=oPitch  DataStoreElements=oPitch.oMot_.oOut_.uiPwmDutyTicksFromMainA_  IndexOptions=Index vector (dialog)  Indices=1  OutputSizes=1
  Data Store Read3 : DataStoreRead  DataStoreName=oPitch  DataStoreElements=oPitch.oMot_.oOut_.uiPwmDutyTicksFromMainB_  IndexOptions=Index vector (dialog)  Indices=1  OutputSizes=1
  Data Store Read5 : DataStoreRead  DataStoreName=oPitch  DataStoreElements=oPitch.oMot_.oOut_.uiPwmDutyTicksFromMainC_  IndexOptions=Index vector (dialog)  Indices=1  OutputSizes=1
  pitchMotor_PWMticks : Outport
  wires:
  Data Store Read3/1 -> Bus Creator2/2  "Bticks"
  Data Store Read5/1 -> Bus Creator2/3  "Cticks"
  Bus Creator2/1 -> pitchMotor_PWMticks/1
  Data Store Read2/1 -> Bus Creator2/1  "Aticks"

== system Target_Control_System/Target_Control_System/MainLoop/pitchMotor_mainLoop/mainTask_pitch/Variant Subsystem/Target_Code_Gen_1/Triggered Subsystem ==
  Trigger : TriggerPort  VariantControl=Variant  InitialTriggerSignalState=zero
  Function-Call Generator : simulink/Ports & Subsystems/Function-Call Generator  sample_time=-1  numberOfIterations=1  DisallowWideOutput=off
  Output : Outport
  wires:
  Function-Call Generator/1 -> Output/1

== system Target_Control_System/Target_Control_System/MainLoop/pitchMotor_mainLoop/mainTask_pitch/motorTaskMainFastStep()/Automatic switching to sensorless - Pitch/Automatic switching to sensorless ==
  note: // Presently disabled, do we need to enable?
  Enable : EnablePort
  Data Store Read2 : DataStoreRead  DataStoreName=oPitch  DataStoreElements=oPitch.oMot_.oState_.fObserverConfidence_  IndexOptions=Index vector (dialog)  Indices=1  OutputSizes=1
  Data Store Read27 : DataStoreRead  DataStoreName=oPitch  DataStoreElements=oPitch.oMot_.oState_.uiSensorlessSwitchoverState_  IndexOptions=Index vector (dialog)  Indices=1  OutputSizes=1
  If : If
  "Switch to sensored " : Subsystem  TreatAsAtomicUnit=on
  Switch to sensorless? : Subsystem  TreatAsAtomicUnit=on
  wires:
  Data Store Read2/1 -> "Switch to sensored "/1(fObserverConfidence), Switch to sensorless?/1(fObserverConfidence)
  Data Store Read27/1 -> If/1
  If/1 -> "Switch to sensored "/Action
  If/2 -> Switch to sensorless?/Action

== system Target_Control_System/Target_Control_System/MainLoop/pitchMotor_mainLoop/mainTask_pitch/motorTaskMainFastStep()/Control Loops - Pitch/Dynamic Current Limiting Pitch ==
  note: // Dynamic current limiting in use
      |       // Behavior:
      |       //  - Integrate the amount the current is over the static limit, squared (because losses scale with I^2R)
      |       //    (Add zero if the current is below the limit)
      |       //  - Apply a leakage factor to the integrator that slowly brings it down to 0. Only if the contribution is zero that time step
      |       //  - Subtract a scaled version of the present integrator value from the dynamic maximum current.
      |       //    (But do not drop below the static maximum)
      |       //
      |       // Actors:
      |       // - opParam->fIqSetpointMax_                       		Static maximum current, in A
      |       // - opParam->fDynILimDynamicMax_                 	Short term maximum current, in A
      |       // - opParam->fDynILimIntegratorLeakageFactor_  Multiplier by which the integrator is multiplied each loop. Examples: 0.1 is very fast bleeddown, 0.999 is alsmost no bleeddown. 1.0 disables bleeddown
      |       // - opParam->fDynILimKnockdownFactor_           	Multiplier by which the integrator is multiplied before subtraction from dynamic_max
      |       // - opStates->fDynILimIntegrator_                  		The integrator state variable
  Enable : EnablePort
  Abs : Abs
  Add : Sum  Inputs=+-
  Add1 : Sum
  Add2 : Sum  Inputs=-+
  Data Store Read : DataStoreRead  DataStoreName=oPitch  DataStoreElements=oPitch.oMot_.oIn_.fIPhaseMagnitude_  IndexOptions=Index vector (dialog)  Indices=1  OutputSizes=1
  Data Store Read1 : DataStoreRead  DataStoreName=oPitch  DataStoreElements=oPitch.oMot_.oParam_.fIqSetpointMax_  IndexOptions=Index vector (dialog)  Indices=1  OutputSizes=1
  Data Store Read10 : DataStoreRead  DataStoreName=oPitch  DataStoreElements=oPitch.oMot_.oParam_.fDynILimIntegratorLeakageFactor_  IndexOptions=Index vector (dialog)  Indices=1  OutputSizes=1
  Data Store Read2 : DataStoreRead  DataStoreName=oPitch  DataStoreElements=oPitch.oMot_.oState_.fDynILimIntegrator_  IndexOptions=Index vector (dialog)  Indices=1  OutputSizes=1
  Data Store Read3 : DataStoreRead  DataStoreName=oPitch  DataStoreElements=oPitch.oMot_.oParam_.fDynILimDynamicMax_  IndexOptions=Index vector (dialog)  Indices=1  OutputSizes=1
  Data Store Read4 : DataStoreRead  DataStoreName=oPitch  DataStoreElements=oPitch.oMot_.oParam_.fTorqueAuthorityFraction_  IndexOptions=Index vector (dialog)  Indices=1  OutputSizes=1
  Data Store Read5 : DataStoreRead  DataStoreName=oPitch  DataStoreElements=oPitch.oMot_.oParam_.fDynILimKnockdownFactor_  IndexOptions=Index vector (dialog)  Indices=1  OutputSizes=1
  Data Store Read6 : DataStoreRead  DataStoreName=oPitch  DataStoreElements=oPitch.oMot_.oState_.fIqRefBeforeRamp_  IndexOptions=Index vector (dialog)  Indices=1  OutputSizes=1
  Data Store Read7 : DataStoreRead  DataStoreName=oPitch  DataStoreElements=oPitch.oMot_.oParam_.fDynILimDynamicMax_  IndexOptions=Index vector (dialog)  Indices=1  OutputSizes=1
  Data Store Write : DataStoreWrite  DataStoreName=oPitch  DataStoreElements=oPitch.oMot_.oState_.fDynILimIntegrator_  IndexOptions=Index vector (dialog)  Indices=1  OutputSizes=1
  Data Store Write1 : DataStoreWrite  DataStoreName=oPitch  DataStoreElements=oPitch.oMot_.oState_.fDynILimActualLimit_  IndexOptions=Index vector (dialog)  Indices=1  OutputSizes=1
  Data Store Write3 : DataStoreWrite  DataStoreName=oPitch  DataStoreElements=oPitch.oMot_.oParam_.oPid2DataRpmCtrl_.oParameter_.fOutMax_  IndexOptions=Index vector (dialog)  Indices=1  OutputSizes=1
  Data Store Write4 : DataStoreWrite  DataStoreName=oPitch  DataStoreElements=oPitch.oMot_.oParam_.oPid2DataRpmCtrl_.oParameter_.fOutMin_  IndexOptions=Index vector (dialog)  Indices=1  OutputSizes=1
  Data Store Write5 : DataStoreWrite  DataStoreName=oPitch  DataStoreElements=oPitch.oMot_.oParam_.oPid2DataRpmCtrl_.oParameter_.fIntMin_  IndexOptions=Index vector (dialog)  Indices=1  OutputSizes=1
  Data Store Write6 : DataStoreWrite  DataStoreName=oPitch  DataStoreElements=oPitch.oMot_.oParam_.oPid2DataRpmCtrl_.oParameter_.fIntMax_  IndexOptions=Index vector (dialog)  Indices=1  OutputSizes=1
  Divide{,1..3} (4 alike) : Product  Inputs=**
  Gain : Gain  Gain=-1
  Gain1 : Gain  Gain=-1
  Gain2 : Gain  Gain=-1
  Max : MinMax  Function=max  Inputs=2
  Max1 : MinMax  Function=max  Inputs=2
  Min : MinMax  Inputs=2
  Switch : Switch  Criteria=u2 > Threshold
  oRampDataIqRef_.fSetpoint : Outport
  wires:
  Gain2/1 -> Data Store Write4/1
  Data Store Read7/1 -> Gain2/1, Data Store Write3/1
  Gain1/1 -> Data Store Write5/1
  Max1/1 -> oRampDataIqRef_.fSetpoint/1
  Gain/1 -> Max1/1
  Min/1 -> Max1/2
  Data Store Read6/1 -> Min/2
  Max/1 -> Min/1, Data Store Write1/1, Gain1/1, Data Store Write6/1, Gain/1
  Add2/1 -> Max/1
  Divide2/1 -> Add2/2
  Divide3/1 -> Add2/1
  Data Store Read5/1 -> Divide3/2
  Data Store Read4/1 -> Divide2/2
  Data Store Read3/1 -> Divide2/1
  Divide1/1 -> Switch/3
  Data Store Read10/1 -> Divide1/2
  Data Store Read2/1 -> Add1/2, Divide1/1
  Divide/1 -> Add1/1
  Switch/1 -> Divide3/1, Data Store Write/1
  Add1/1 -> Switch/1
  Add/1 -> Switch/2, Divide/2, Divide/1  "fTemp"
  Abs/1 -> Add/1
  Data Store Read1/1 -> Add/2, Max/2
  Data Store Read/1 -> Abs/1

== system Target_Control_System/Target_Control_System/MainLoop/pitchMotor_mainLoop/mainTask_pitch/motorTaskMainFastStep()/Control Loops - Pitch/Flux Weakening - Pitch ==
  Constant : Constant  Value=0  OutDataTypeStr=single  SampleTime=-1
  oRampDataIdRef_.fSetpoint : Outport
  wires:
  Constant/1 -> oRampDataIdRef_.fSetpoint/1
